simulink subsystem "Ultrasonic_System_Simulation_ThorneFleissner"  (R2020b)
settings: Solver=VariableStepAuto  StartTime=0.0  StopTime=10.0  RelTol=1e-3
settings Model: Creator=rthom  LastModifiedBy=rthom

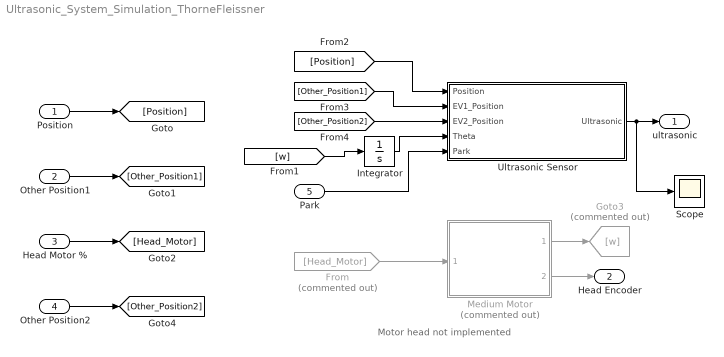
== system Ultrasonic_System_Simulation_ThorneFleissner ==
  note: Motor head not implemented
  Position : Inport
  Other Position1 : Inport  Port=2
  Head Motor % : Inport  Port=3
  Other Position2 : Inport  Port=4
  Park : Inport  Port=5
  From : From  Commented=on  GotoTag=Head_Motor
  Goto3 : Goto  Commented=on  GotoTag=w
  Integrator : Integrator
  Medium Motor : Subsystem  Commented=on  ReferencedSubsystem=Medium_Motor_ThorneFleissner
  Scope : Scope
  Ultrasonic Sensor : MATLAB Function  TreatAsAtomicUnit=on  SystemSampleTime=0.05
  ultrasonic : Outport
  Head Encoder : Outport  Port=2
  wires:
  Position/1 -> [Position]
  Head Motor %/1 -> [Head_Motor]
  Other Position1/1 -> [Other_Position1]
  From/1 -> Medium Motor/1
  Ultrasonic Sensor/1(Ultrasonic) -> ultrasonic/1, Scope/1
  Medium Motor/1 -> Goto3/1
  Medium Motor/2 -> Head Encoder/1
  [Other_Position1] -> Ultrasonic Sensor/2(EV1_Position)
  [Position] -> Ultrasonic Sensor/1(Position)
  [w] -> Integrator/1
  Integrator/1 -> Ultrasonic Sensor/4(Theta)
  [Other_Position2] -> Ultrasonic Sensor/3(EV2_Position)
  Other Position2/1 -> [Other_Position2]
  Park/1 -> Ultrasonic Sensor/5(Park)

== matlab function Ultrasonic_System_Simulation_ThorneFleissner/Ultrasonic Sensor ==
  data: Position input; Ultrasonic output; EV1_Position input; EV2_Position input; Theta input; Park input
function Ultrasonic = UltrasonicFcn(Position,EV1_Position,EV2_Position,Theta,Park)
%% Parking Spot Position Constants
    Spot1_Up = [-1.308; 0.9163];
    Spot1_Down = [-1.3115; 0.6954];
    Spot2_Up = [-1.1672; 1.3082];
    Spot2_Down = [-1.1647; 1.0837];
    Spot3_Up = [-0.8906; 1.72];
    Spot3_Down = [-0.8977; 1.5883];

    Spot1_Mid = (Spot1_Up(1:2)+ Spot1_Down(1:2))/2;
    Spot2_Mid = (Spot2_Up(1:2)+ Spot2_Down(1:2))/2;
    Spot3_Mid = (Spot3_Up(1:2)+ Spot3_Down(1:2))/2;

%% Other EV 1
    %Calculate the position between the objects
        EV1_Distance_XZ = EV1_Position(1:2) - Position(1:2);%Calculating the x and z values for the distance between the EV's
        EV1_Distance_Hypot = sqrt((EV1_Distance_XZ(1)^2)+(EV1_Distance_XZ(2)^2));%Calculating hypotenuse using calculated x and z values
        EV1_Distance_Hypot = (EV1_Distance_Hypot*100) - 14;%Convert from m to cm and move points from center of EVs to back of other EV (7cm) and front of EV (7cm) NOTE: 7cm is from center of brick to front of brick, shouldn't it be to the front of the sensor?
    
    %Adjust Boundary of Sensor based on Distance
       
        EV1_Base_Boundary = 50;%Define the base boundary value
        
        if EV1_Distance_Hypot <= 60 && EV1_Distance_Hypot >= 30
          EV1_Boundary = EV1_Base_Boundary + 10; 
        elseif EV1_Distance_Hypot<=30 && EV1_Distance_Hypot>=20
          EV1_Boundary = EV1_Base_Boundary + 20; 
        elseif EV1_Distance_Hypot<20
          EV1_Boundary = EV1_Base_Boundary + 30;
        else
          EV1_Boundary = EV1_Base_Boundary;
        end
        
    %Calculate Desired Angle of Ultrasonic Sensor
        EV1_alpha_rad = atan2(EV1_Distance_XZ(2),EV1_Distance_XZ(1)) - Position(3);%Radians, Calculating the desired head angle of the ultrasonic sensor in relation to the EV body
        EV1_alpha_deg = rad2deg(EV1_alpha_rad);%Convert alpha from radians to degrees
        EV1_alpha_desired = mod(EV1_alpha_deg + 180, 360) - 180;%Limit the desired head angle betweeen -180 and 180 deg
        
    %Range Boundary Calculations
        EV1_boundary_pos = EV1_alpha_desired + EV1_Boundary;%Calculate positive boundary
        EV1_boundary_pos = mod(EV1_boundary_pos + 180, 360) - 180;%Limit boundary between -180 and 180
        EV1_boundary_neg = EV1_alpha_desired - EV1_Boundary;%Calculate negative boundary
        EV1_boundary_neg = mod(EV1_boundary_neg + 180, 360) - 180;%Limit boundary between -180 and 180
        
%% Other EV 2
    %Calculate the position between the objects
        EV2_Distance_XZ = EV2_Position(1:2) - Position(1:2);%Calculating the x and z values for the distance between the EV's
        EV2_Distance_Hypot = sqrt((EV2_Distance_XZ(1)^2)+(EV2_Distance_XZ(2)^2));%Calculating hypotenuse using calculated x and z values
        EV2_Distance_Hypot = (EV2_Distance_Hypot*100) - 14;%Convert from m to cm and move points from center of EVs to back of other EV (7cm) and front of EV (7cm) NOTE: 7cm is from center of brick to front of brick, shouldn't it be to the front of the sensor?
    
    %Adjust Boundary of Sensor based on Distance
       
        EV2_Base_Boundary = 50;%Define the base boundary value
        
        if EV2_Distance_Hypot <= 60 && EV2_Distance_Hypot >= 30
          EV2_Boundary = EV2_Base_Boundary + 10; 
        elseif EV2_Distance_Hypot<=30 && EV2_Distance_Hypot>=20
          EV2_Boundary = EV2_Base_Boundary + 20; 
        elseif EV2_Distance_Hypot<20
          EV2_Boundary = EV2_Base_Boundary + 30;
        else
          EV2_Boundary = EV2_Base_Boundary;
        end
        
    %Calculate Desired Angle of Ultrasonic Sensor
        EV2_alpha_rad = atan2(EV2_Distance_XZ(2),EV2_Distance_XZ(1)) - Position(3);%Radians, Calculating the desired head angle of the ultrasonic sensor in relation to the EV body
        EV2_alpha_deg = rad2deg(EV2_alpha_rad);%Convert alpha from radians to degrees
        EV2_alpha_desired = mod(EV2_alpha_deg + 180, 360) - 180;%Limit the desired head angle betweeen -180 and 180 deg
        
    %Range Boundary Calculations
        EV2_boundary_pos = EV2_alpha_desired + EV2_Boundary;%Calculate positive boundary
        EV2_boundary_pos = mod(EV2_boundary_pos + 180, 360) - 180;%Limit boundary between -180 and 180
        EV2_boundary_neg = EV2_alpha_desired - EV2_Boundary;%Calculate negative boundary
        EV2_boundary_neg = mod(EV2_boundary_neg + 180, 360) - 180;%Limit boundary between -180 and 180
        
%% Parking Spot 1
    %Calculate the position between the objects
        Spot1_Distance_XZ = Spot1_Mid(1:2) - Position(1:2);%Calculating the x and z values for the distance between the EV and parking spot 1
        Spot1_Distance_Hypot = sqrt((Spot1_Distance_XZ(1)^2)+(Spot1_Distance_XZ(2)^2));%Calculating hypotenuse using calculated x and z values
        Spot1_Distance_Hypot = (Spot1_Distance_Hypot*100) - 7;%Convert from m to cm and move distance to front of EV (NOTE: should probably be front of sensor not EV)

     %Adjust Boundary of Sensor based on Distance
       
        Spot1_Base_Boundary = 10;%Define the base boundary value
        
        if Spot1_Distance_Hypot <= 60 && Spot1_Distance_Hypot >= 30
          Spot1_Boundary = Spot1_Base_Boundary + 10; 
        elseif Spot1_Distance_Hypot<=30 && Spot1_Distance_Hypot>=20
          Spot1_Boundary = Spot1_Base_Boundary + 20; 
        elseif Spot1_Distance_Hypot<20
          Spot1_Boundary = Spot1_Base_Boundary + 30;
        else
          Spot1_Boundary = Spot1_Base_Boundary;
        end
        
    %Calculate Desired Angle of Ultrasonic Sensor
        Spot1_alpha_rad = atan2(Spot1_Distance_XZ(2),Spot1_Distance_XZ(1)) - Position(3);%Radians, Calculating the desired head angle of the ultrasonic sensor in relation to the EV body
        Spot1_alpha_deg = rad2deg(Spot1_alpha_rad);%Convert alpha from radians to degrees
        Spot1_alpha_desired = mod(Spot1_alpha_deg + 180, 360) - 180;%Limit the desired head angle betweeen -180 and 180 deg
        
    %Range Boundary Calculations
        Spot1_boundary_pos = Spot1_alpha_desired + Spot1_Boundary;%Calculate positive boundary
        Spot1_boundary_pos = mod(Spot1_boundary_pos + 180, 360) - 180;%Limit boundary between -180 and 180
        Spot1_boundary_neg = Spot1_alpha_desired - Spot1_Boundary;%Calculate negative boundary
        Spot1_boundary_neg = mod(Spot1_boundary_neg + 180, 360) - 180;%Limit boundary between -180 and 180
        
%% Parking Spot 2
    %Calculate the position between the objects
        Spot2_Distance_XZ = Spot2_Mid(1:2) - Position(1:2);%Calculating the x and z values for the distance between the EV and parking spot 2
        Spot2_Distance_Hypot = sqrt((Spot2_Distance_XZ(1)^2)+(Spot2_Distance_XZ(2)^2));%Calculating hypotenuse using calculated x and z values
        Spot2_Distance_Hypot = (Spot2_Distance_Hypot*100) - 7;%Convert from m to cm and move distance to front of EV (NOTE: should probably be front of sensor not EV)
        
     %Adjust Boundary of Sensor based on Distance
       
        Spot2_Base_Boundary = 10;%Define the base boundary value
        
        if Spot2_Distance_Hypot <= 60 && Spot2_Distance_Hypot >= 30
          Spot2_Boundary = Spot2_Base_Boundary + 10; 
        elseif Spot2_Distance_Hypot<=30 && Spot2_Distance_Hypot>=20
          Spot2_Boundary = Spot2_Base_Boundary + 20; 
        elseif Spot2_Distance_Hypot<20
          Spot2_Boundary = Spot2_Base_Boundary + 30; 
        else
          Spot2_Boundary = Spot2_Base_Boundary;
        end
        
    %Calculate Desired Angle of Ultrasonic Sensor
        Spot2_alpha_rad = atan2(Spot2_Distance_XZ(2),Spot2_Distance_XZ(1)) - Position(3);%Radians, Calculating the desired head angle of the ultrasonic sensor in relation to the EV body
        Spot2_alpha_deg = rad2deg(Spot2_alpha_rad);%Convert alpha from radians to degrees
        Spot2_alpha_desired = mod(Spot2_alpha_deg + 180, 360) - 180;%Limit the desired head angle betweeen -180 and 180 deg
        
    %Range Boundary Calculations
        Spot2_boundary_pos = Spot2_alpha_desired + Spot2_Boundary;%Calculate positive boundary
        Spot2_boundary_pos = mod(Spot2_boundary_pos + 180, 360) - 180;%Limit boundary between -180 and 180
        Spot2_boundary_neg = Spot2_alpha_desired - Spot2_Boundary;%Calculate negative boundary
        Spot2_boundary_neg = mod(Spot2_boundary_neg + 180, 360) - 180;%Limit boundary between -180 and 180
        
%% Parking Spot 3
    %Calculate the position between the objects
        Spot3_Distance_XZ = Spot3_Mid(1:2) - Position(1:2);%Calculating the x and z values for the distance between the EV and parking spot 3
        Spot3_Distance_Hypot = sqrt((Spot3_Distance_XZ(1)^2)+(Spot3_Distance_XZ(2)^2));%Calculating hypotenuse using calculated x and z values
        Spot3_Distance_Hypot = (Spot3_Distance_Hypot*100) - 7;%Convert from m to cm and move distance to front of EV (NOTE: should probably be front of sensor not EV)
        
     %Adjust Boundary of Sensor based on Distance
       
        Spot3_Base_Boundary = 10;%Define the base boundary value
        
        if Spot3_Distance_Hypot <= 60 && Spot3_Distance_Hypot >= 30
          Spot3_Boundary = Spot3_Base_Boundary + 10; 
        elseif Spot3_Distance_Hypot<=30 && Spot3_Distance_Hypot>=20
          Spot3_Boundary = Spot3_Base_Boundary + 20; 
        elseif Spot3_Distance_Hypot<20
          Spot3_Boundary = Spot3_Base_Boundary + 30; 
        else
          Spot3_Boundary = Spot3_Base_Boundary;
        end
        
    %Calculate Desired Angle of Ultrasonic Sensor
        Spot3_alpha_rad = atan2(Spot3_Distance_XZ(2),Spot3_Distance_XZ(1)) - Position(3);%Radians, Calculating the desired head angle of the ultrasonic sensor in relation to the EV body
        Spot3_alpha_deg = rad2deg(Spot3_alpha_rad);%Convert alpha from radians to degrees
        Spot3_alpha_desired = mod(Spot3_alpha_deg + 180, 360) - 180;%Limit the desired head angle betweeen -180 and 180 deg
        
    %Range Boundary Calculations
        Spot3_boundary_pos = Spot3_alpha_desired + Spot3_Boundary;%Calculate positive boundary
        Spot3_boundary_pos = mod(Spot3_boundary_pos + 180, 360) - 180;%Limit boundary between -180 and 180
        Spot3_boundary_neg = Spot3_alpha_desired - Spot3_Boundary;%Calculate negative boundary
        Spot3_boundary_neg = mod(Spot3_boundary_neg + 180, 360) - 180;%Limit boundary between -180 and 180
        
%% Calculate Ultrasonic Output
    %Calculate Actual Angle of Ultrasonic Sensor
        theta_deg = rad2deg(Theta);%Convert theta from radians to degrees
        theta_actual = mod(theta_deg + 180, 360) - 180;%Limit the actual head angle between -180 and 180 deg
    %Determine Which Distance to Use if within Motor Head Boundary
        Ultrasonic = 255;%cm, Set the default value of the ultrasonic sensor to the maximum output
        
        if (((EV1_boundary_neg <= theta_actual) && (EV1_boundary_pos >= theta_actual)) && (EV1_boundary_pos > EV1_boundary_neg)) ...
            || (~((EV1_boundary_pos <= theta_actual) && (EV1_boundary_neg >= theta_actual)) && (EV1_boundary_neg >= EV1_boundary_pos))
                Ultrasonic = min(Ultrasonic, EV1_Distance_Hypot);
                
        elseif (((EV2_boundary_neg <= theta_actual) && (EV2_boundary_pos >= theta_actual)) && (EV2_boundary_pos > EV2_boundary_neg)) ...
            || (~((EV2_boundary_pos <= theta_actual) && (EV2_boundary_neg >= theta_actual)) && (EV2_boundary_neg >= EV2_boundary_pos))
                Ultrasonic = min(Ultrasonic, EV2_Distance_Hypot);
                
        elseif Park == 1 && (((Spot1_boundary_neg <= theta_actual) && (Spot1_boundary_pos >= theta_actual)) && (Spot1_boundary_pos > Spot1_boundary_neg)) ...
            || (~((Spot1_boundary_pos <= theta_actual) && (Spot1_boundary_neg >= theta_actual)) && (Spot1_boundary_neg >= Spot1_boundary_pos))
                Ultrasonic = min(Ultrasonic, Spot1_Distance_Hypot);
                
        elseif Park == 1 && (((Spot2_boundary_neg <= theta_actual) && (Spot2_boundary_pos >= theta_actual)) && (Spot2_boundary_pos > Spot2_boundary_neg)) ...
            || (~((Spot2_boundary_pos <= theta_actual) && (Spot2_boundary_neg >= theta_actual)) && (Spot2_boundary_neg >= Spot2_boundary_pos))
                Ultrasonic = min(Ultrasonic, Spot2_Distance_Hypot);
                
        elseif Park == 1 && (((Spot3_boundary_neg <= theta_actual) && (Spot3_boundary_pos >= theta_actual)) && (Spot3_boundary_pos > Spot3_boundary_neg)) ...
            || (~((Spot3_boundary_pos <= theta_actual) && (Spot3_boundary_neg >= theta_actual)) && (Spot3_boundary_neg >= Spot3_boundary_pos))
                Ultrasonic = min(Ultrasonic, Spot3_Distance_Hypot);
        end
end
